simulink model "testIntegral"  (R2012b)
settings: Solver=ode45  StartTime=0.0  StopTime=10.0  RelTol=1e-3
undefined symbols (not defined in the file or in its folder): DiscIntNeverNeededParam
libraries: WBCLibrary x2, utility x1
settings Model: Creator=daniele  LastModifiedBy=daniele

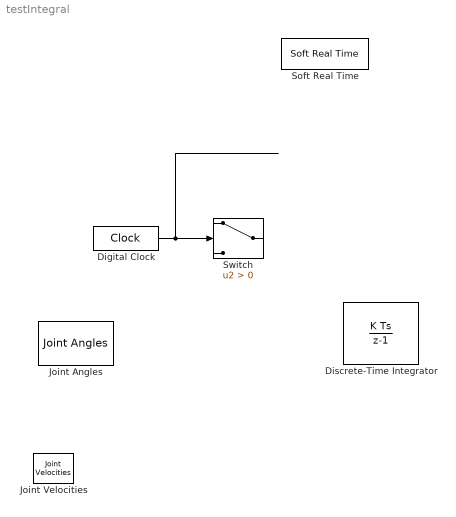
== system testIntegral ==
  Digital Clock : DigitalClock  SampleTime=-1
  Discrete-Time Integrator : DiscreteIntegrator  SampleTime=0.01  ICPrevOutput=DiscIntNeverNeededParam  ICPrevScaledInput=DiscIntNeverNeededParam
  Joint Angles : WBCLibrary/wholeBodyStates/Joint Angles  robotName=robotName  localName=localName
  Joint Velocities : WBCLibrary/wholeBodyStates/Joint Velocities  robotName=robotName  localName=localName
  Soft Real Time : utility/Soft Real Time  x=0.01
  Switch : Switch  Criteria=u2 > Threshold
  wires:
  Digital Clock/1 -> Switch/2
